simulink library "SOMANETHandler"  (R2016b)
settings: Solver=VariableStepAuto  StartTime=0.0  StopTime=10.0  RelTol=1e-3
undefined symbols (not defined in the file or in its folder): SomanetError
libraries: VariousLibrary x18, SOMANET x5
settings Model: Creator=Nathan  LastModifiedBy=march

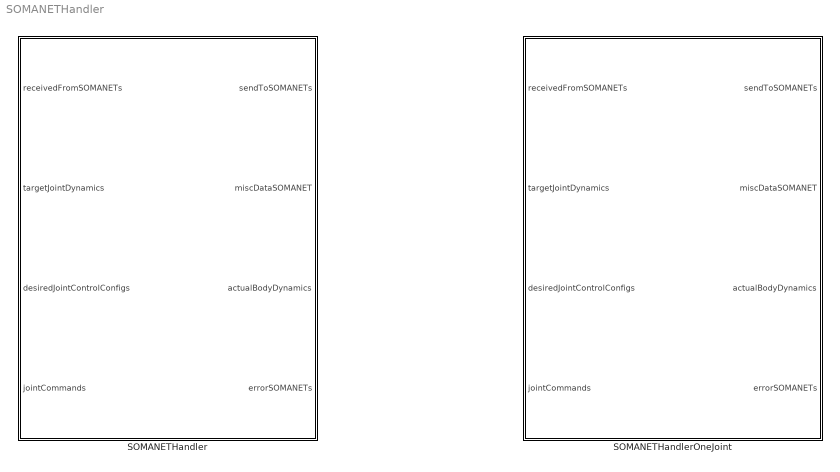
== system SOMANETHandler ==
  SOMANETHandler : Subsystem
  SOMANETHandlerOneJoint : Subsystem  AncestorBlock=SOMANETHandler/SOMANETHandler

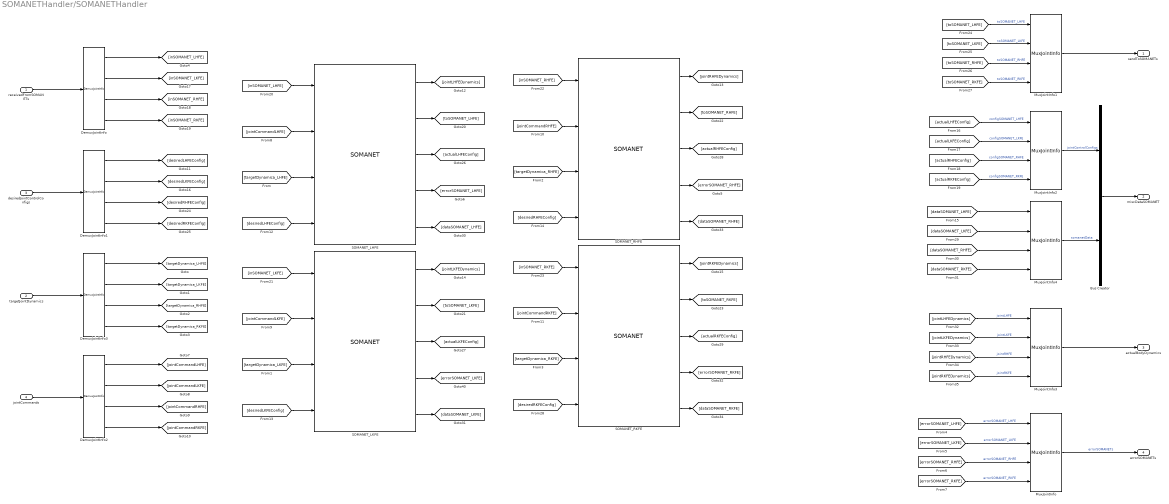
== system SOMANETHandler/SOMANETHandler ==
  receivedFromSOMANETs : Inport  OutDataTypeStr=Bus: EtherCATReceivedFromSOMANET  PortDimensions=[1 4]  BusOutputAsStruct=on
  targetJointDynamics : Inport  Port=2  OutDataTypeStr=Bus: JointDynamics  PortDimensions=[1 4]
  desiredJointControlConfigs : Inport  Port=3  OutDataTypeStr=Bus: JointControlConfig  PortDimensions=[1 4]
  jointCommands : Inport  Port=4
  Bus Creator : BusCreator  Inputs=2  OutDataTypeStr=Bus: MiscDataSOMANET  NonVirtualBus=on
  DemuxJointInfo{,1..3} (4 alike) : VariousLibrary/DemuxJointInfo
  MuxJointInfo{,1..4} (5 alike) : VariousLibrary/MuxJointInfo
  SOMANET_LHFE : SOMANET/SOMANET
  SOMANET_LKFE : SOMANET/SOMANET
  SOMANET_RHFE : SOMANET/SOMANET
  SOMANET_RKFE : SOMANET/SOMANET
  sendToSOMANETs : Outport  OutDataTypeStr=Bus: EtherCATSendToSOMANET  PortDimensions=[1 4]  BusOutputAsStruct=on
  miscDataSOMANET : Outport  Port=2
  actualBodyDynamics : Outport  Port=3
  errorSOMANETs : Outport  Port=4  OutDataTypeStr=Enum: SomanetError  PortDimensions=[1 4]  BusOutputAsStruct=on
  wires:
  jointCommands/1 -> DemuxJointInfo2/1
  DemuxJointInfo2/4 -> [jointCommandRKFE]
  DemuxJointInfo2/3 -> [jointCommandRHFE]
  DemuxJointInfo2/1 -> [jointCommandLHFE]
  DemuxJointInfo2/2 -> [jointCommandLKFE]
  DemuxJointInfo3/1 -> [targetDynamica_LHFE]
  DemuxJointInfo3/2 -> [targetDynamica_LKFE]
  DemuxJointInfo3/3 -> [targetDynamica_RHFE]
  DemuxJointInfo3/4 -> [targetDynamica_RKFE]
  MuxJointInfo4/1 -> Bus Creator/2  "somanetData"
  MuxJointInfo2/1 -> Bus Creator/1  "jointControlConfigs"
  [dataSOMANET_RKFE] -> MuxJointInfo4/4
  [dataSOMANET_RHFE] -> MuxJointInfo4/3
  [dataSOMANET_LKFE] -> MuxJointInfo4/2
  [dataSOMANET_LHFE] -> MuxJointInfo4/1
  SOMANET_RKFE/5 -> [dataSOMANET_RKFE]
  SOMANET_RHFE/5 -> [dataSOMANET_RHFE]
  SOMANET_LKFE/5 -> [dataSOMANET_LKFE]
  SOMANET_LHFE/5 -> [dataSOMANET_LHFE]
  [errorSOMANET_LKFE] -> MuxJointInfo/2  "errorSOMANET_LKFE"
  [errorSOMANET_RKFE] -> MuxJointInfo/4  "errorSOMANET_RKFE"
  [errorSOMANET_RHFE] -> MuxJointInfo/3  "errorSOMANET_RHFE"
  [errorSOMANET_LHFE] -> MuxJointInfo/1  "errorSOMANET_LHFE"
  MuxJointInfo/1 -> errorSOMANETs/1  "errorSOMANETs"
  [targetDynamica_RKFE] -> SOMANET_RKFE/3
  [targetDynamica_RHFE] -> SOMANET_RHFE/3
  [targetDynamica_LKFE] -> SOMANET_LKFE/3
  [toSOMANET_RHFE] -> MuxJointInfo1/3  "toSOMANET_RHFE"
  [toSOMANET_RKFE] -> MuxJointInfo1/4  "toSOMANET_RKFE"
  [toSOMANET_LKFE] -> MuxJointInfo1/2  "toSOMANET_LKFE"
  [inSOMANET_RKFE] -> SOMANET_RKFE/1
  [actualLKFEConfig] -> MuxJointInfo2/2  "configSOMANET_LKFE"
  [actualLHFEConfig] -> MuxJointInfo2/1  "configSOMANET_LHFE"
  [toSOMANET_LHFE] -> MuxJointInfo1/1  "toSOMANET_LHFE"
  MuxJointInfo1/1 -> sendToSOMANETs/1
  [inSOMANET_RHFE] -> SOMANET_RHFE/1
  [inSOMANET_LKFE] -> SOMANET_LKFE/1
  [inSOMANET_LHFE] -> SOMANET_LHFE/1
  [actualRKFEConfig] -> MuxJointInfo2/4  "configSOMANET_RKFE"
  [actualRHFEConfig] -> MuxJointInfo2/3  "configSOMANET_RHFE"
  Bus Creator/1 -> miscDataSOMANET/1
  SOMANET_RHFE/1 -> [jointRHFEDynamics]
  SOMANET_LKFE/1 -> [jointLKFEDynamics]
  SOMANET_RKFE/1 -> [jointRKFEDynamics]
  SOMANET_RHFE/2 -> [toSOMANET_RHFE]
  SOMANET_RHFE/3 -> [actualRHFEConfig]
  SOMANET_RHFE/4 -> [errorSOMANET_RHFE]
  SOMANET_RKFE/2 -> [toSOMANET_RKFE]
  SOMANET_RKFE/3 -> [actualRKFEConfig]
  SOMANET_RKFE/4 -> [errorSOMANET_RKFE]
  SOMANET_LKFE/2 -> [toSOMANET_LKFE]
  SOMANET_LKFE/3 -> [actualLKFEConfig]
  SOMANET_LKFE/4 -> [errorSOMANET_LKFE]
  [jointLHFEDynamics] -> MuxJointInfo3/1  "jointLHFE"
  [jointLKFEDynamics] -> MuxJointInfo3/2  "jointLKFE"
  [jointRHFEDynamics] -> MuxJointInfo3/3  "jointRHFE"
  [jointRKFEDynamics] -> MuxJointInfo3/4  "jointRKFE"
  MuxJointInfo3/1 -> actualBodyDynamics/1
  [jointCommandLHFE] -> SOMANET_LHFE/2
  [jointCommandLKFE] -> SOMANET_LKFE/2
  [jointCommandRHFE] -> SOMANET_RHFE/2
  [jointCommandRKFE] -> SOMANET_RKFE/2
  desiredJointControlConfigs/1 -> DemuxJointInfo1/1
  DemuxJointInfo1/4 -> [desiredRKFEConfig]
  DemuxJointInfo1/3 -> [desiredRHFEConfig]
  DemuxJointInfo1/2 -> [desiredLKFEConfig]
  DemuxJointInfo1/1 -> [desiredLHFEConfig]
  [desiredLKFEConfig] -> SOMANET_LKFE/4
  [desiredRHFEConfig] -> SOMANET_RHFE/4
  [desiredRKFEConfig] -> SOMANET_RKFE/4
  receivedFromSOMANETs/1 -> DemuxJointInfo/1
  DemuxJointInfo/4 -> [inSOMANET_RKFE]
  DemuxJointInfo/2 -> [inSOMANET_LKFE]
  DemuxJointInfo/3 -> [inSOMANET_RHFE]
  DemuxJointInfo/1 -> [inSOMANET_LHFE]
  [desiredLHFEConfig] -> SOMANET_LHFE/4
  [targetDynamica_LHFE] -> SOMANET_LHFE/3
  SOMANET_LHFE/1 -> [jointLHFEDynamics]
  SOMANET_LHFE/2 -> [toSOMANET_LHFE]
  SOMANET_LHFE/3 -> [actualLHFEConfig]
  SOMANET_LHFE/4 -> [errorSOMANET_LHFE]
  targetJointDynamics/1 -> DemuxJointInfo3/1

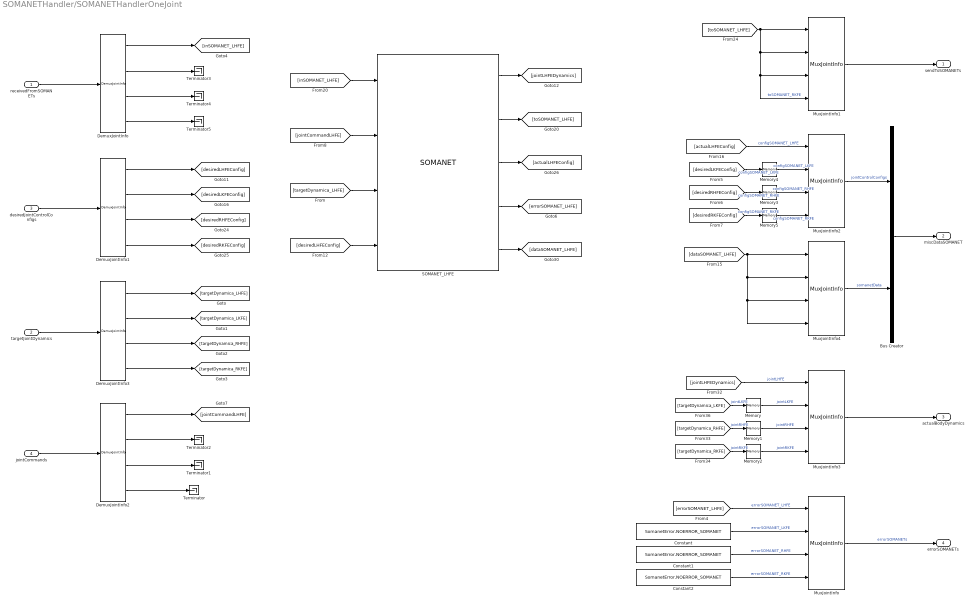
== system SOMANETHandler/SOMANETHandlerOneJoint ==
  receivedFromSOMANETs : Inport  OutDataTypeStr=Bus: EtherCATReceivedFromSOMANET  PortDimensions=[1 4]  BusOutputAsStruct=on
  targetJointDynamics : Inport  Port=2  OutDataTypeStr=Bus: JointDynamics  PortDimensions=[1 4]
  desiredJointControlConfigs : Inport  Port=3  OutDataTypeStr=Bus: JointControlConfig  PortDimensions=[1 4]
  jointCommands : Inport  Port=4
  Bus Creator : BusCreator  Inputs=2  OutDataTypeStr=Bus: MiscDataSOMANET  NonVirtualBus=on
  Constant : Constant  Value=SomanetError.NOERROR_SOMANET
  Constant1 : Constant  Value=SomanetError.NOERROR_SOMANET
  Constant2 : Constant  Value=SomanetError.NOERROR_SOMANET
  DemuxJointInfo{,1..3} (4 alike) : VariousLibrary/DemuxJointInfo
  Memory{,1..5} (6 alike) : Memory
  MuxJointInfo{,1..4} (5 alike) : VariousLibrary/MuxJointInfo
  SOMANET_LHFE : SOMANET/SOMANET
  Terminator{,1..5} (6 alike) : Terminator
  sendToSOMANETs : Outport  OutDataTypeStr=Bus: EtherCATSendToSOMANET  PortDimensions=[1 4]  BusOutputAsStruct=on
  miscDataSOMANET : Outport  Port=2
  actualBodyDynamics : Outport  Port=3
  errorSOMANETs : Outport  Port=4  OutDataTypeStr=Enum: SomanetError  PortDimensions=[1 4]  BusOutputAsStruct=on
  wires:
  jointCommands/1 -> DemuxJointInfo2/1
  DemuxJointInfo2/4 -> Terminator/1
  DemuxJointInfo2/3 -> Terminator1/1
  DemuxJointInfo2/1 -> [jointCommandLHFE]
  DemuxJointInfo2/2 -> Terminator2/1
  DemuxJointInfo3/1 -> [targetDynamica_LHFE]
  DemuxJointInfo3/2 -> [targetDynamica_LKFE]
  DemuxJointInfo3/3 -> [targetDynamica_RHFE]
  DemuxJointInfo3/4 -> [targetDynamica_RKFE]
  MuxJointInfo4/1 -> Bus Creator/2  "somanetData"
  MuxJointInfo2/1 -> Bus Creator/1  "jointControlConfigs"
  [dataSOMANET_LHFE] -> MuxJointInfo4/1, MuxJointInfo4/3, MuxJointInfo4/4, MuxJointInfo4/2
  SOMANET_LHFE/5 -> [dataSOMANET_LHFE]
  Constant/1 -> MuxJointInfo/2  "errorSOMANET_LKFE"
  Constant2/1 -> MuxJointInfo/4  "errorSOMANET_RKFE"
  Constant1/1 -> MuxJointInfo/3  "errorSOMANET_RHFE"
  [errorSOMANET_LHFE] -> MuxJointInfo/1  "errorSOMANET_LHFE"
  MuxJointInfo/1 -> errorSOMANETs/1  "errorSOMANETs"
  [toSOMANET_LHFE] -> MuxJointInfo1/1, MuxJointInfo1/2, MuxJointInfo1/3, MuxJointInfo1/4  "toSOMANET_RKFE"
  Memory4/1 -> MuxJointInfo2/2  "configSOMANET_LKFE"
  [actualLHFEConfig] -> MuxJointInfo2/1  "configSOMANET_LHFE"
  MuxJointInfo1/1 -> sendToSOMANETs/1
  [inSOMANET_LHFE] -> SOMANET_LHFE/1
  Memory3/1 -> MuxJointInfo2/3  "configSOMANET_RHFE"
  Bus Creator/1 -> miscDataSOMANET/1
  [jointLHFEDynamics] -> MuxJointInfo3/1  "jointLHFE"
  Memory/1 -> MuxJointInfo3/2  "jointLKFE"
  Memory1/1 -> MuxJointInfo3/3  "jointRHFE"
  Memory2/1 -> MuxJointInfo3/4  "jointRKFE"
  MuxJointInfo3/1 -> actualBodyDynamics/1
  [jointCommandLHFE] -> SOMANET_LHFE/2
  desiredJointControlConfigs/1 -> DemuxJointInfo1/1
  DemuxJointInfo1/4 -> [desiredRKFEConfig]
  DemuxJointInfo1/3 -> [desiredRHFEConfig]
  DemuxJointInfo1/2 -> [desiredLKFEConfig]
  DemuxJointInfo1/1 -> [desiredLHFEConfig]
  receivedFromSOMANETs/1 -> DemuxJointInfo/1
  DemuxJointInfo/4 -> Terminator5/1
  DemuxJointInfo/2 -> Terminator3/1
  DemuxJointInfo/3 -> Terminator4/1
  DemuxJointInfo/1 -> [inSOMANET_LHFE]
  [desiredLHFEConfig] -> SOMANET_LHFE/4
  [targetDynamica_LHFE] -> SOMANET_LHFE/3
  SOMANET_LHFE/1 -> [jointLHFEDynamics]
  SOMANET_LHFE/2 -> [toSOMANET_LHFE]
  SOMANET_LHFE/3 -> [actualLHFEConfig]
  SOMANET_LHFE/4 -> [errorSOMANET_LHFE]
  targetJointDynamics/1 -> DemuxJointInfo3/1
  [targetDynamica_LKFE] -> Memory/1  "jointLKFE"
  [targetDynamica_RKFE] -> Memory2/1  "jointRKFE"
  [targetDynamica_RHFE] -> Memory1/1  "jointRHFE"
  [desiredLKFEConfig] -> Memory4/1  "configSOMANET_LKFE"
  [desiredRHFEConfig] -> Memory3/1  "configSOMANET_RHFE"
  [desiredRKFEConfig] -> Memory5/1  "configSOMANET_RKFE"
  Memory5/1 -> MuxJointInfo2/4  "configSOMANET_RKFE"
